simulink model "cycletest_feedback"  (R2023a)
settings: Solver=ode1  StartTime=0  StopTime=1200  FixedStep=0.002  RelTol=1e-3  EnableMultiTasking=on
values from neighbouring files (symbols this model uses):
  cycleGain = 0.2    [simulate_hover.m]    (also in temp.m = 1)
  Jp = 2*Jeq_prop    (= 0.0552224595625)    [setup_lab_hover.m]    (also in simulate_hover.m)
  Jr = 2*Jeq_prop    (= 0.0552224595625)    [setup_lab_hover.m]    (also in simulate_hover.m)
  Jy = 4*Jeq_prop    (= 0.110444919125)    [setup_lab_hover.m]    (also in simulate_hover.m)
  K = lqi(sys, Q, R)    [simulate_hover.m]
  kd = 0.5    [simulate_hover.m]
  Kf = 0.1188    [setup_lab_hover.m]    (also in simulate_hover.m)
  Kt = 0.0036    [setup_lab_hover.m]    (also in simulate_hover.m)
  L = 7.75*0.0254    (= 0.19685)    [setup_lab_hover.m]    (also in simulate_hover.m = 0.1969)
  r = flexSize(no)    [phaseComp.m]    (also in simulate_hover.m = 0.5)
  sigma = 0    [simulate_hover.m]
  skew = 2    [simulate_hover.m]
  V_bias = 12    [setup_lab_hover.m]    (also in simulate_hover.m)
  VMAX_AMP = 24    [setup_lab_hover.m]    (also in simulate_hover.m)
  wcf = 2 * pi * 20    (= 125.663706144)    [setup_lab_hover.m]    (also in simulate_hover.m)
  zetaf = 0.6    [setup_lab_hover.m]    (also in simulate_hover.m)
libraries: simulink_extras x4, dspsrcs4 x1
settings Model: ExtModeTrigDuration=10000  Creator=kille  LastModifiedBy=Jacob
settings SolverCC: AlgebraicLoopSolver=TrustRegion  PositivePriorityOrder=on  AutoInsertRateTranBlk=on
settings DataIOCC: ReturnWorkspaceOutputs=off
settings OptimizationCC: LifeSpan=inf
settings DebuggingCC: UnconnectedInputMsg=warning  UnconnectedOutputMsg=warning  UnconnectedLineMsg=warning  ArithmeticOperatorsInVariantConditions=warning
settings ModelReferenceCC: EnableRefExpFcnMdlSchedulingChecks=on
settings SFSimCC: SimUseLocalCustomCode=off  CustomCodeUndefinedFunction=UseInterfaceOnly
settings RTWCC: Description=QUARC Win64 Target  SystemTargetFile=quarc_win64.tlc  TemplateMakefile=quarc_default_tmf  RTWUseLocalCustomCode=off
settings CodeAppCC: StateflowObjectComments=on
settings STFCustomTargetCC: TargetPreCompLibLocation=C:\PROGRA~3\QUARC\lib\2016a\win64\release  UseToolchainInfoCompliant=off  SystemTargetFile=quarc_win64.tlc
settings GRTTargetCC: TargetPreCompLibLocation=C:\PROGRA~3\QUARC\lib\2016a\win64\release  ParMdlRefBuildCompliant=off  CompOptLevelCompliant=off  CombineOutputUpdateFcns=off  MatFileLogging=off  CPPClassGenCompliant=off  GRTInterface=on  UseToolchainInfoCompliant=off  ExtMode=on  ExtModeMexFile=quarc_comm
settings ConfigComp: CovMetricSettings=dswe

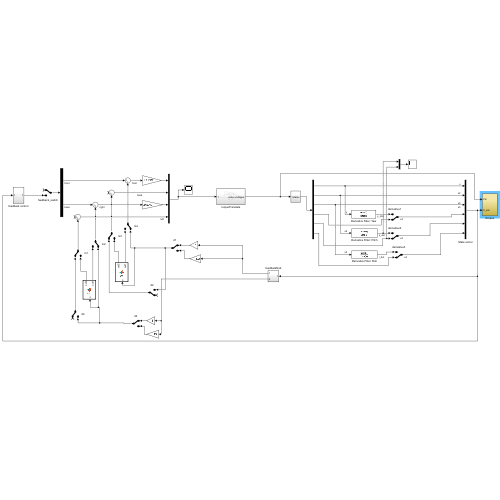
[thumbnail: Simulink's stored preview of the top-level diagram]
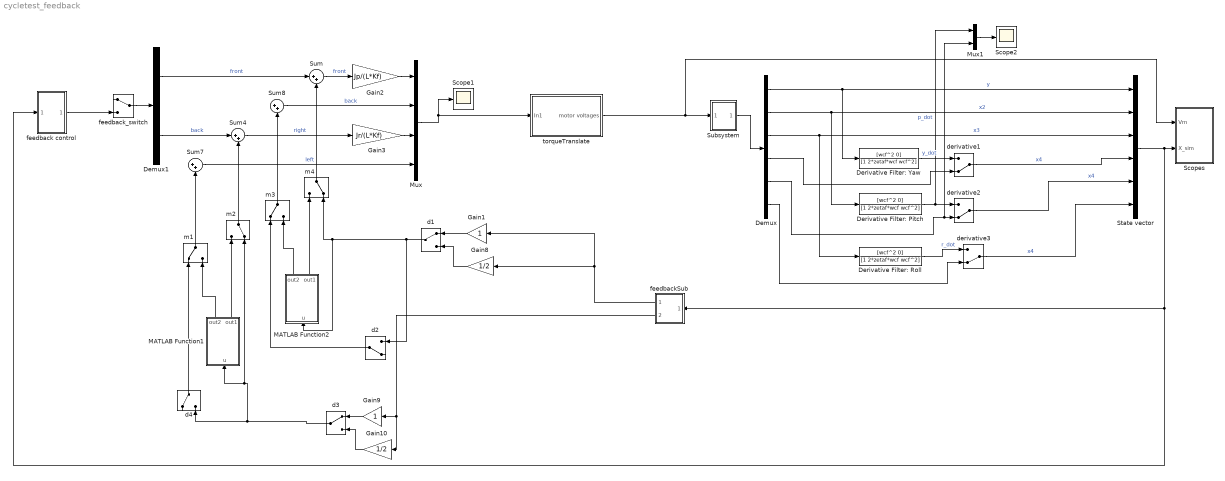
== system cycletest_feedback ==
  Demux : Demux  Outputs=6
  Demux1 : Demux  Outputs=2
  Derivative Filter: Pitch : TransferFcn  Numerator=[wcf^2 0]  Denominator=[1 2*zetaf*wcf wcf^2]
  Derivative Filter: Roll : TransferFcn  Numerator=[wcf^2 0]  Denominator=[1 2*zetaf*wcf wcf^2]
  Derivative Filter: Yaw : TransferFcn  Numerator=[wcf^2 0]  Denominator=[1 2*zetaf*wcf wcf^2]
  Gain1 : Gain
  Gain10 : Gain  Gain=1/2
  Gain2 : Gain  Gain=Jp/(L*Kf)
  Gain3 : Gain  Gain=Jr/(L*Kf)
  Gain8 : Gain  Gain=1/2
  Gain9 : Gain
  MATLAB Function1 : MATLAB Function  TreatAsAtomicUnit=on
  MATLAB Function2 : MATLAB Function  TreatAsAtomicUnit=on
  Mux : Mux
  Mux1 : Mux  Inputs=2
  Scope1 : Scope
  Scope2 : Scope
  Scopes : Subsystem
  State vector : Mux  Inputs=6
  Subsystem : Subsystem
  Sum{,4,7..8} (4 alike) : Sum  Inputs=|++
  d1 : ManualSwitch
  d2 : ManualSwitch  CurrentSetting=0
  d3 : ManualSwitch
  d4 : ManualSwitch
  derivative1 : ManualSwitch  CurrentSetting=0
  derivative2 : ManualSwitch  CurrentSetting=0
  derivative3 : ManualSwitch  CurrentSetting=0
  feedback control : Subsystem
  feedbackSub : Subsystem
  feedback_switch : ManualSwitch
  m1 : ManualSwitch
  m2 : ManualSwitch  CurrentSetting=0
  m3 : ManualSwitch
  m4 : ManualSwitch  CurrentSetting=0
  torqueTranslate : Subsystem
  wires:
  Demux/1 -> State vector/1, Derivative Filter: Yaw/1  "y"
  m2/1 -> Sum4/2
  m3/1 -> Sum8/2
  m4/1 -> Sum/2
  m1/1 -> Sum7/2
  Sum7/1 -> Mux/4  "left"
  Sum8/1 -> Mux/2  "back"
  Mux/1 -> torqueTranslate/1(In1), Scope1/1
  MATLAB Function2/2(out1) -> m4/1
  MATLAB Function2/1(out2) -> m3/2
  MATLAB Function1/2(out1) -> m2/1
  MATLAB Function1/1(out2) -> m1/2
  Derivative Filter: Yaw/1 -> derivative1/1  "y_dot"
  Demux/4 -> derivative1/2
  Derivative Filter: Pitch/1 -> Mux1/1, derivative2/1  "p_dot"
  Derivative Filter: Roll/1 -> derivative3/1  "r_dot"
  Demux/5 -> Mux1/2, derivative2/2
  Demux/6 -> derivative3/2
  derivative1/1 -> State vector/4  "x4"
  derivative3/1 -> State vector/6  "x4"
  Demux/3 -> State vector/3, Derivative Filter: Roll/1  "x3"
  Demux/2 -> State vector/2, Derivative Filter: Pitch/1  "x2"
  feedbackSub/1(Out1) -> Gain8/1, Gain1/1
  Gain1/1 -> d1/1
  Gain8/1 -> d1/2
  d1/1 -> d2/1, m4/2, MATLAB Function2/1(u)
  d2/1 -> m3/1
  feedbackSub/2(Out2) -> Gain10/1, Gain9/1
  Gain9/1 -> d3/1
  d3/1 -> MATLAB Function1/1(u), m2/2, d4/2
  Gain10/1 -> d3/2
  d4/1 -> m1/1
  feedback_switch/1 -> Demux1/1
  State vector/1 -> feedbackSub/1(Input), feedback control/1(In1), Scopes/2(X_sim)
  Demux1/1 -> Sum/1  "front"
  Demux1/2 -> Sum4/1  "back"
  Subsystem/1(states) -> Demux/1
  Sum/1 -> Gain2/1  "front"
  Sum4/1 -> Gain3/1  "right"
  torqueTranslate/1(motor voltages) -> Scopes/1(Vm), Subsystem/1(Input)
  Mux1/1 -> Scope2/1
  Gain2/1 -> Mux/1
  Gain3/1 -> Mux/3
  feedback control/1(Out1) -> feedback_switch/2
  derivative2/1 -> State vector/5  "x4"

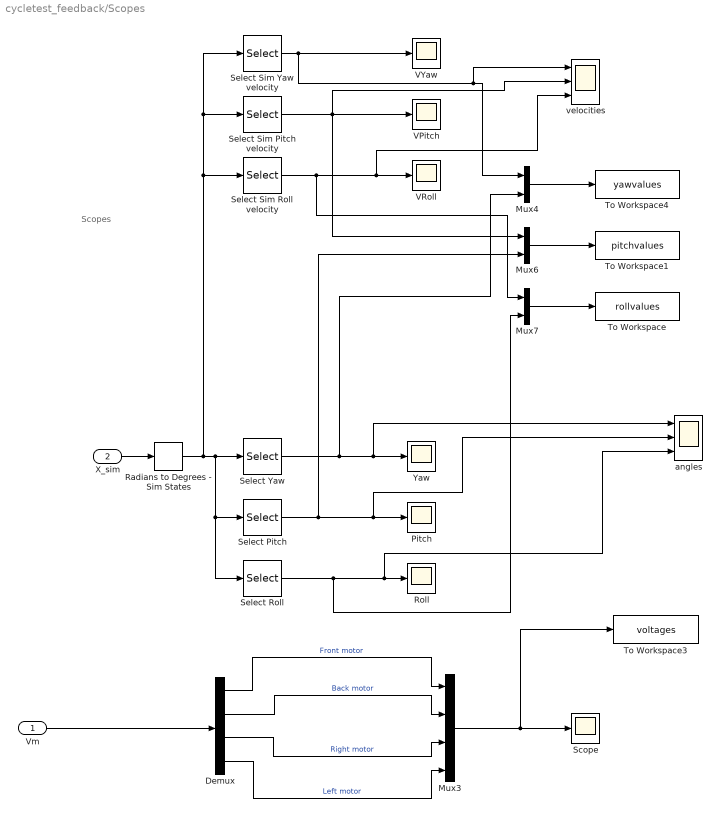
== system cycletest_feedback/Scopes ==
  note: Scopes
  Vm : Inport
  X_sim : Inport  Port=2
  Demux : Demux
  Mux3 : Mux
  Mux4 : Mux  Inputs=2
  Mux6 : Mux  Inputs=2
  Mux7 : Mux  Inputs=2
  Pitch : Scope
  Radians to Degrees - Sim States : simulink_extras/Transformations/Radians to Degrees
  Roll : Scope
  Scope : Scope
  Select Pitch : Selector  InputPortWidth=6  IndexOptions=Index vector (dialog)  Indices=2  OutputSizes=1
  Select Roll : Selector  InputPortWidth=6  IndexOptions=Index vector (dialog)  Indices=3  OutputSizes=1
  Select Sim Pitch velocity : Selector  InputPortWidth=6  IndexOptions=Index vector (dialog)  Indices=5  OutputSizes=1
  Select Sim Roll velocity : Selector  InputPortWidth=6  IndexOptions=Index vector (dialog)  Indices=6  OutputSizes=1
  Select Sim Yaw velocity : Selector  InputPortWidth=6  IndexOptions=Index vector (dialog)  Indices=4  OutputSizes=1
  Select Yaw : Selector  InputPortWidth=6  IndexOptions=Index vector (dialog)  Indices=1  OutputSizes=1
  To Workspace : ToWorkspace  VariableName=rollvalues  SampleTime=-1
  To Workspace1 : ToWorkspace  VariableName=pitchvalues  SampleTime=-1
  To Workspace3 : ToWorkspace  VariableName=voltages  SampleTime=-1
  To Workspace4 : ToWorkspace  VariableName=yawvalues  SampleTime=-1
  VPitch : Scope
  VRoll : Scope
  VYaw : Scope
  Yaw : Scope
  angles : Scope  NumInputPorts=3
  velocities : Scope  NumInputPorts=3
  wires:
  Select Roll/1 -> angles/3, Roll/1, Mux7/2
  Radians to Degrees - Sim States/1 -> Select Sim Roll velocity/1, Select Sim Pitch velocity/1, Select Sim Yaw velocity/1, Select Roll/1, Select Pitch/1, Select Yaw/1
  Select Pitch/1 -> angles/2, Pitch/1, Mux6/2
  X_sim/1 -> Radians to Degrees - Sim States/1
  Demux/1 -> Mux3/1  "Front motor"
  Demux/2 -> Mux3/2  "Back motor"
  Demux/3 -> Mux3/3  "Right motor"
  Demux/4 -> Mux3/4  "Left motor"
  Vm/1 -> Demux/1
  Select Sim Yaw velocity/1 -> VYaw/1, velocities/1, Mux4/1
  Select Sim Roll velocity/1 -> velocities/3, VRoll/1, Mux7/1
  Select Sim Pitch velocity/1 -> Mux6/1, velocities/2, VPitch/1
  Mux4/1 -> To Workspace4/1
  Mux6/1 -> To Workspace1/1
  Mux7/1 -> To Workspace/1
  Mux3/1 -> To Workspace3/1, Scope/1
  Select Yaw/1 -> angles/1, Yaw/1, Mux4/2

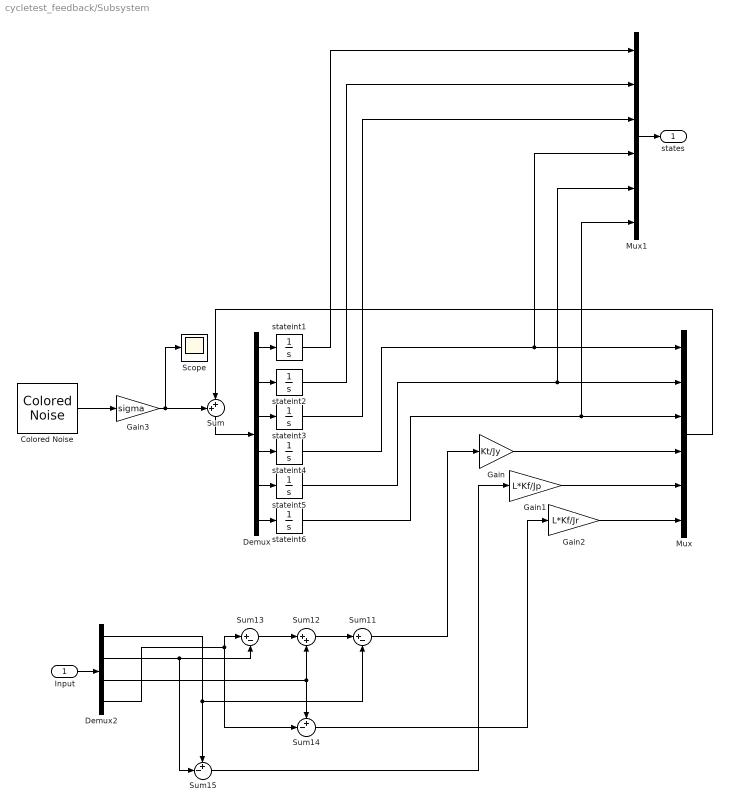
== system cycletest_feedback/Subsystem ==
  Input : Inport
  Colored Noise : dspsrcs4/Colored Noise  Color=white  InverseFrequencyPower=1  BoundedOutput=off  NumChannels=6  OutputDataType=double  SamplesPerFrame=1  SampleTime=1  RandomStream=mt19937ar with seed  Seed=67  SimulateUsing=Interpreted execution
  Demux : Demux  Outputs=6
  Demux2 : Demux
  Gain : Gain  Gain=Kt/Jy
  Gain1 : Gain  Gain=L*Kf/Jp
  Gain2 : Gain  Gain=L*Kf/Jr
  Gain3 : Gain  Gain=sigma
  Mux : Mux  Inputs=6
  Mux1 : Mux  Inputs=6
  Scope : Scope
  Sum : Sum  Inputs=++|
  Sum11 : Sum  Inputs=|+-
  Sum12 : Sum  Inputs=|++
  Sum13 : Sum  Inputs=|+-
  Sum14 : Sum  Inputs=+-|
  Sum15 : Sum  Inputs=+-|
  stateint1 : Integrator  InitialCondition=0.017453
  stateint2 : Integrator  InitialCondition=0.017453
  stateint3 : Integrator  InitialCondition=0.017453
  stateint4 : Integrator
  stateint5 : Integrator
  stateint6 : Integrator
  states : Outport
  wires:
  stateint5/1 -> Mux/2, Mux1/5
  Gain2/1 -> Mux/6
  Gain1/1 -> Mux/5
  stateint6/1 -> Mux/3, Mux1/6
  stateint4/1 -> Mux/1, Mux1/4
  Gain/1 -> Mux/4
  Mux/1 -> Sum/2
  Gain3/1 -> Scope/1, Sum/1
  Demux2/4 -> Sum13/1, Sum14/2
  Demux2/1 -> Sum15/1, Sum11/2
  Demux2/2 -> Sum13/2, Sum15/2
  Sum12/1 -> Sum11/1
  Sum11/1 -> Gain/1
  Demux2/3 -> Sum12/2, Sum14/1
  Sum13/1 -> Sum12/1
  Input/1 -> Demux2/1
  Sum/1 -> Demux/1
  Demux/1 -> stateint1/1
  Demux/2 -> stateint2/1
  Demux/3 -> stateint3/1
  Demux/4 -> stateint4/1
  Demux/5 -> stateint5/1
  Demux/6 -> stateint6/1
  Mux1/1 -> states/1
  stateint1/1 -> Mux1/1
  stateint2/1 -> Mux1/2
  stateint3/1 -> Mux1/3
  Sum15/1 -> Gain1/1
  Sum14/1 -> Gain2/1
  Colored Noise/1 -> Gain3/1

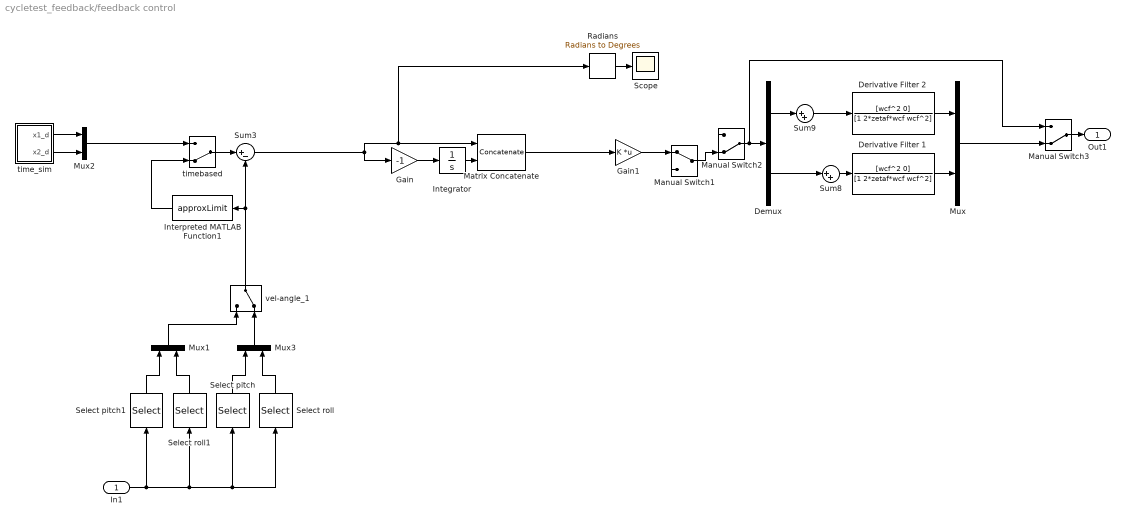
== system cycletest_feedback/feedback control ==
  In1 : Inport
  Demux : Demux  Outputs=2
  Derivative Filter 1 : TransferFcn  Numerator=[wcf^2 0]  Denominator=[1 2*zetaf*wcf wcf^2]
  Derivative Filter 2 : TransferFcn  Numerator=[wcf^2 0]  Denominator=[1 2*zetaf*wcf wcf^2]
  Gain : Gain  Gain=-1
  Gain1 : Gain  Gain=K  Multiplication=Matrix(K*u)
  Integrator : Integrator
  Interpreted MATLAB Function1 : MATLABFcn  MATLABFcn=approxLimit  Output1D=off
  Manual Switch1 : ManualSwitch
  Manual Switch2 : ManualSwitch  CurrentSetting=0
  Manual Switch3 : ManualSwitch  CurrentSetting=0
  Matrix Concatenate : Concatenate  Mode=Multidimensional array
  Mux{,1..3} (4 alike) : Mux  Inputs=2
  Radians : simulink_extras/Transformations/Radians to Degrees
  Scope : Scope
  Select pitch : Selector  InputPortWidth=6  IndexOptions=Index vector (dialog)  Indices=2  OutputSizes=1
  Select pitch1 : Selector  InputPortWidth=6  IndexOptions=Index vector (dialog)  Indices=5  OutputSizes=1
  Select roll : Selector  InputPortWidth=6  IndexOptions=Index vector (dialog)  Indices=3  OutputSizes=1
  Select roll1 : Selector  InputPortWidth=6  IndexOptions=Index vector (dialog)  Indices=6  OutputSizes=1
  Sum3 : Sum  Inputs=|+-
  Sum8 : Sum  Inputs=|++
  Sum9 : Sum  Inputs=|++
  time_sim : Subsystem
  timebased : ManualSwitch  CurrentSetting=0
  vel-angle_1 : ManualSwitch  CurrentSetting=0
  Out1 : Outport
  wires:
  time_sim/1(x1_d) -> Mux2/1
  time_sim/2(x2_d) -> Mux2/2
  Select pitch/1 -> Mux3/1
  In1/1 -> Select roll1/1, Select roll/1, Select pitch/1, Select pitch1/1
  Mux3/1 -> vel-angle_1/2
  Mux1/1 -> vel-angle_1/1
  Select roll/1 -> Mux3/2
  Select roll1/1 -> Mux1/2
  Select pitch1/1 -> Mux1/1
  Manual Switch1/1 -> Manual Switch2/2
  Demux/1 -> Sum9/1
  Derivative Filter 2/1 -> Mux/1
  Sum9/1 -> Derivative Filter 2/1
  Manual Switch3/1 -> Out1/1
  Derivative Filter 1/1 -> Mux/2
  Demux/2 -> Sum8/1
  Sum8/1 -> Derivative Filter 1/1
  Mux/1 -> Manual Switch3/2
  Radians/1 -> Scope/1
  Manual Switch2/1 -> Manual Switch3/1, Demux/1
  Interpreted MATLAB Function1/1 -> timebased/2
  vel-angle_1/1 -> Sum3/2, Interpreted MATLAB Function1/1
  Mux2/1 -> timebased/1
  timebased/1 -> Sum3/1
  Gain/1 -> Integrator/1
  Integrator/1 -> Matrix Concatenate/2
  Matrix Concatenate/1 -> Gain1/1
  Gain1/1 -> Manual Switch1/1
  Sum3/1 -> Gain/1, Radians/1, Matrix Concatenate/1

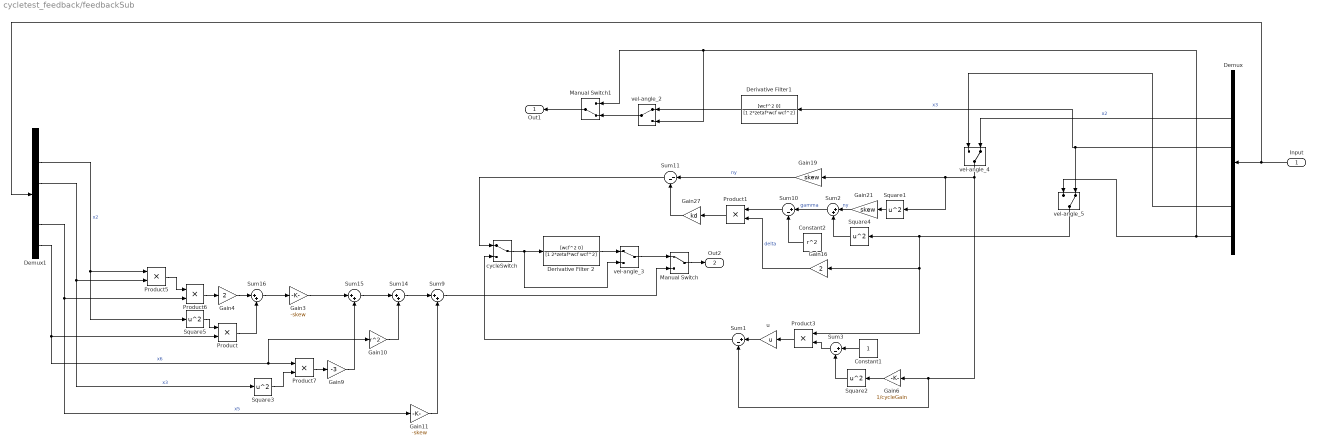
== system cycletest_feedback/feedbackSub ==
  Input : Inport
  Constant1 : Constant
  Constant2 : Constant  Value=r^2
  Demux : Demux  Outputs=6
  Demux1 : Demux  Outputs=6
  Derivative Filter 2 : TransferFcn  Numerator=[wcf^2 0]  Denominator=[1 2*zetaf*wcf wcf^2]
  Derivative Filter1 : TransferFcn  Numerator=[wcf^2 0]  Denominator=[1 2*zetaf*wcf wcf^2]
  Gain10 : Gain  Gain=r^2
  Gain11 : Gain  Gain=-skew
  Gain16 : Gain  Gain=2
  Gain19 : Gain  Gain=skew
  Gain21 : Gain  Gain=skew
  Gain27 : Gain  Gain=kd
  Gain3 : Gain  Gain=-skew
  Gain4 : Gain  Gain=2
  Gain6 : Gain  Gain=1/cycleGain
  Gain9 : Gain  Gain=-3
  Manual Switch : ManualSwitch
  Manual Switch1 : ManualSwitch  CurrentSetting=0
  Product{,1,3,5..7} (6 alike) : Product
  Square{1..5} (5 alike) : Math  Operator=square
  Sum1 : Sum  Inputs=|+-
  Sum10 : Sum  Inputs=|+-
  Sum11 : Sum  Inputs=|--
  Sum{2,9,14..16} (5 alike) : Sum  Inputs=|++
  Sum3 : Sum  Inputs=|+-
  cycleSwitch : ManualSwitch
  u : Gain  Gain=u
  vel-angle_2 : ManualSwitch
  vel-angle_3 : ManualSwitch
  vel-angle_4 : ManualSwitch  CurrentSetting=0
  vel-angle_5 : ManualSwitch  CurrentSetting=0
  Out1 : Outport
  Out2 : Outport  Port=2
  wires:
  Square1/1 -> Gain21/1
  Product1/1 -> Gain27/1
  Square4/1 -> Sum2/2
  Gain19/1 -> Sum11/1  "ny"
  Sum2/1 -> Sum10/1  "gamma"
  Gain16/1 -> Product1/2  "delta"
  Sum10/1 -> Product1/1
  Gain27/1 -> Sum11/2
  Gain21/1 -> Sum2/1  "ny"
  Constant2/1 -> Sum10/2
  Sum1/1 -> cycleSwitch/2
  Demux/3 -> Derivative Filter1/1, vel-angle_5/2  "x3"
  u/1 -> Sum1/1
  Gain6/1 -> Square2/1
  Product3/1 -> u/1
  Constant1/1 -> Sum3/1
  Sum3/1 -> Product3/2
  Square2/1 -> Sum3/2
  Demux/2 -> vel-angle_4/2  "x2"
  Sum11/1 -> cycleSwitch/1
  Derivative Filter1/1 -> vel-angle_2/1
  Derivative Filter 2/1 -> vel-angle_3/1
  Input/1 -> Demux1/1, Demux/1
  vel-angle_4/1 -> Gain6/1, Sum1/2, Square1/1, Gain19/1
  Demux/5 -> vel-angle_4/1
  vel-angle_5/1 -> Product3/1, Gain16/1, Square4/1
  Demux/6 -> vel-angle_2/2, Manual Switch1/1, vel-angle_5/1
  cycleSwitch/1 -> Derivative Filter 2/1, vel-angle_3/2
  Product6/1 -> Gain4/1
  Demux1/3 -> Square3/1, Product5/2  "x3"
  Gain10/1 -> Sum14/2
  Product5/1 -> Product6/1
  Gain11/1 -> Sum9/2
  Gain4/1 -> Sum16/1
  Square3/1 -> Product7/2
  Gain9/1 -> Sum15/2
  Sum16/1 -> Gain3/1
  Product/1 -> Sum16/2
  Demux1/2 -> Product5/1, Square5/1  "x2"
  Sum15/1 -> Sum14/1
  Gain3/1 -> Sum15/1
  Square5/1 -> Product/1
  Sum14/1 -> Sum9/1
  Demux1/5 -> Gain11/1, Product6/2  "x5"
  Demux1/6 -> Gain10/1, Product7/1, Product/2  "x6"
  Product7/1 -> Gain9/1
  vel-angle_3/1 -> Manual Switch/1
  Manual Switch/1 -> Out2/1
  Sum9/1 -> Manual Switch/2
  vel-angle_2/1 -> Manual Switch1/2
  Manual Switch1/1 -> Out1/1

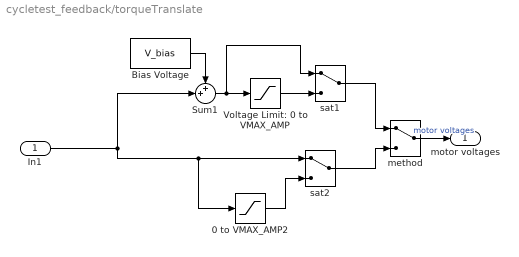
== system cycletest_feedback/torqueTranslate ==
  In1 : Inport
  0 to VMAX_AMP2 : Saturate  UpperLimit=VMAX_AMP  LowerLimit=0
  Bias Voltage : Constant  Value=V_bias
  Sum1 : Sum  Inputs=++|
  Voltage Limit: 0 to VMAX_AMP : Saturate  UpperLimit=VMAX_AMP  LowerLimit=0
  method : ManualSwitch  Tag=swt
  sat1 : ManualSwitch
  sat2 : ManualSwitch
  motor voltages : Outport
  wires:
  sat2/1 -> method/2
  In1/1 -> 0 to VMAX_AMP2/1, sat2/1, Sum1/2
  Bias Voltage/1 -> Sum1/1
  Sum1/1 -> sat1/1, Voltage Limit: 0 to VMAX_AMP/1
  Voltage Limit: 0 to VMAX_AMP/1 -> sat1/2
  method/1 -> motor voltages/1  "motor voltages"
  0 to VMAX_AMP2/1 -> sat2/2
  sat1/1 -> method/1

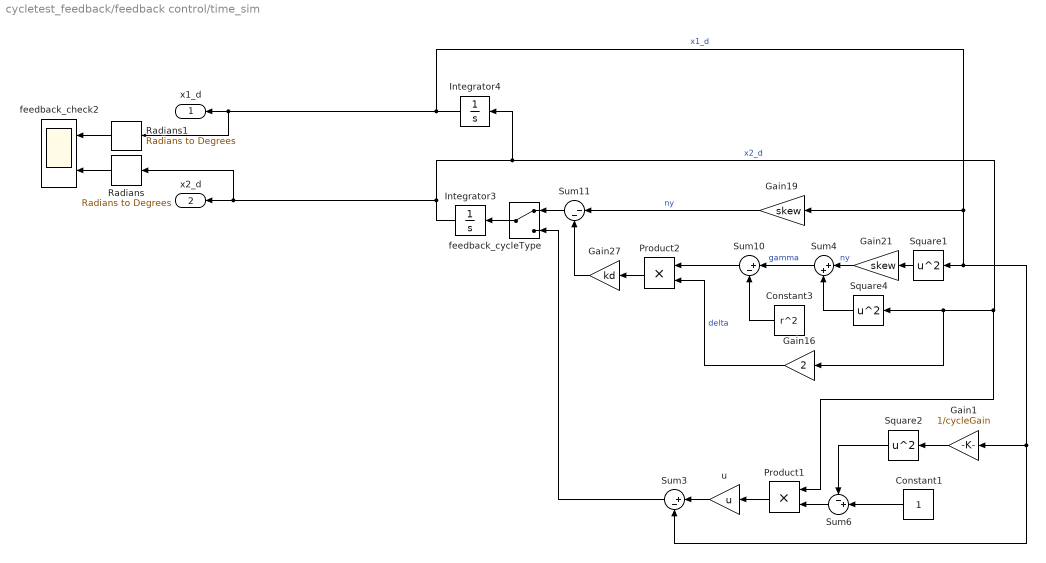
== system cycletest_feedback/feedback control/time_sim ==
  Constant1 : Constant
  Constant3 : Constant  Value=r^2
  Gain1 : Gain  Gain=1/cycleGain
  Gain16 : Gain  Gain=2
  Gain19 : Gain  Gain=skew
  Gain21 : Gain  Gain=skew
  Gain27 : Gain  Gain=kd
  Integrator3 : Integrator  InitialCondition=0.00010472
  Integrator4 : Integrator  InitialCondition=0.00010472
  Product1 : Product
  Product2 : Product
  Radians : simulink_extras/Transformations/Radians to Degrees
  Radians1 : simulink_extras/Transformations/Radians to Degrees
  Square1 : Math  Operator=square
  Square2 : Math  Operator=square
  Square4 : Math  Operator=square
  Sum10 : Sum  Inputs=|+-
  Sum11 : Sum  Inputs=|--
  Sum3 : Sum  Inputs=|+-
  Sum4 : Sum  Inputs=|++
  Sum6 : Sum  Inputs=-+|
  feedback_check2 : Scope  NumInputPorts=2
  feedback_cycleType : ManualSwitch
  u : Gain  Gain=u
  x1_d : Outport
  x2_d : Outport  Port=2
  wires:
  Square1/1 -> Gain21/1
  Square4/1 -> Sum4/2
  Integrator4/1 -> Sum3/2, Gain1/1, Square1/1, Gain19/1, Radians1/1, x1_d/1  "x1_d"
  Gain27/1 -> Sum11/2
  Gain16/1 -> Product2/2  "delta"
  Gain19/1 -> Sum11/1  "ny"
  Integrator3/1 -> Product1/1, Gain16/1, Square4/1, Integrator4/1, Radians/1, x2_d/1  "x2_d"
  Sum10/1 -> Product2/1
  Constant3/1 -> Sum10/2
  Gain21/1 -> Sum4/1  "ny"
  Sum4/1 -> Sum10/1  "gamma"
  Product2/1 -> Gain27/1
  Radians1/1 -> feedback_check2/1
  Radians/1 -> feedback_check2/2
  Square2/1 -> Sum6/1
  Gain1/1 -> Square2/1
  u/1 -> Sum3/1
  Product1/1 -> u/1
  Sum6/1 -> Product1/2
  Constant1/1 -> Sum6/2
  feedback_cycleType/1 -> Integrator3/1
  Sum11/1 -> feedback_cycleType/1
  Sum3/1 -> feedback_cycleType/2

== matlab function cycletest_feedback/MATLAB Function2 ==
  data: out2 output; u input; out1 output
function [out2, out1] = fcn(u)

if u > 0
    out1 = u;
    out2 = 0;
else
    out1 = 0;
    out2 = -u;
end

== matlab function cycletest_feedback/MATLAB Function1 ==
  data: out2 output; u input; out1 output
function [out2, out1] = fcn(u)

if u > 0
    out1 = u;
    out2 = 0;
else
    out1 = 0;
    out2 = -u;
end
